simulink model "PID_cont_single"  (R2013a)
settings: Solver=ode45  StartTime=0.0  StopTime=5  FixedStep=0.00001  RelTol=1e-3
libraries: simulink x1
settings Model: Creator=Brandon  LastModifiedBy=Brandon
settings SolverCC: ZeroCrossAlgorithm=Adaptive

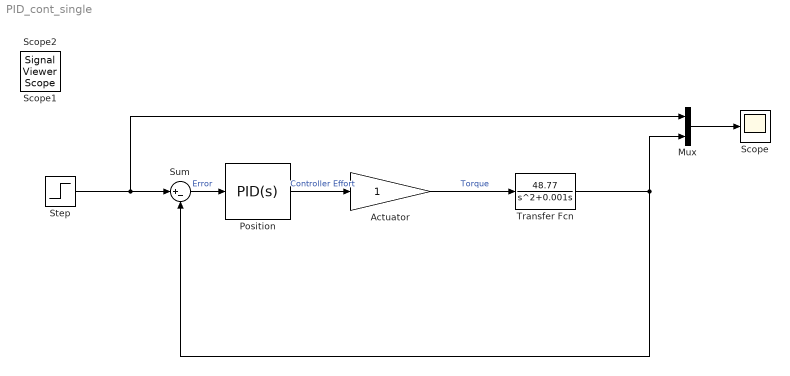
== system PID_cont_single ==
  Actuator : Gain
  Mux : Mux  Inputs=2
  "Position " : simulink/Continuous/PID Controller  Controller=PID  TimeDomain=Continuous-time  SampleTime=0.01  IntegratorMethod=Forward Euler  FilterMethod=Forward Euler  Form=Ideal  P=0.817064877586056  I=0.227315388448101  D=0.977444561139097  N=4452.95769102796  InitialConditionSource=internal  InitialConditionForIntegrator=0  InitialConditionForFilter=0  ExternalReset=none  LimitOutput=off  UpperSaturationLimit=10  LowerSaturationLimit=-10  LinearizeAsGain=on  AntiWindupMode=clamping  Kb=1  TrackingMode=off  Kt=1  PParamMin=[]  PParamMax=[]  IParamMin=[]  IParamMax=[]  DParamMin=[]  DParamMax=[]  NParamMin=[]  NParamMax=[]  KbParamMin=[]  KbParamMax=[]  KtParamMin=[]  KtParamMax=[]  POutMin=[]  POutMax=[]  IOutMin=[]  IOutMax=[]  DOutMin=[]  DOutMax=[]  NOutMin=[]  NOutMax=[]  KbOutMin=[]  KbOutMax=[]  KtOutMin=[]  KtOutMax=[]  IntegratorOutMin=[]  IntegratorOutMax=[]  FilterOutMin=[]  FilterOutMax=[]  SumOutMin=[]  SumOutMax=[]  SumI1OutMin=[]  SumI1OutMax=[]  SumI2OutMin=[]  SumI2OutMax=[]  SumI3OutMin=[]  SumI3OutMax=[]  SumDOutMin=[]  SumDOutMax=[]  SaturationOutMin=[]  SaturationOutMax=[]  IntegratorContinuousStateAttributes=''  IntegratorStateMustResolveToSignalObject=off  IntegratorRTWStateStorageClass=Auto  FilterContinuousStateAttributes=''  FilterStateMustResolveToSignalObject=off  FilterRTWStateStorageClass=Auto
      link override Filter: IntegratorMethod=Integration: Forward Euler  gainval=1.0  ExternalReset=none  InitialConditionSource=internal  InitialCondition=InitialConditionForFilter  InitialConditionMode=State only (most efficient)  SampleTime=-1  OutMin=FilterOutMin  OutMax=FilterOutMax  OutDataTypeStr=FilterOutDataTypeStr  LimitOutput=off  UpperSaturationLimit=inf  LowerSaturationLimit=-inf  ShowSaturationPort=off  ShowStatePort=off
      link override Filter: StateMustResolveToSignalObject=off  RTWStateStorageClass=Auto
  Scope : Scope
      settings: TimeRange=5
  Step : Step
  Sum : Sum  Inputs=|+-
  Transfer Fcn : TransferFcn  Numerator=[48.77]  Denominator=[1 0.001 0 ]
  Scope1 : SignalViewerScope  IOType=viewer  ZoomMode=yonly  RefreshTime=0.035000
  Scope2 : SignalViewerScope  IOType=viewer  ZoomMode=yonly  RefreshTime=0.035000
      settings: SaveName=ScopeData2
  wires:
  Step/1 -> Mux/1, Sum/1
  Transfer Fcn/1 -> Sum/2, Mux/2
  Sum/1 -> "Position "/1  "Error"
  Actuator/1 -> Transfer Fcn/1  "Torque"
  Mux/1 -> Scope/1
  "Position "/1 -> Actuator/1  "Controller Effort"
